simulink model "BTL"  (R2019b)
settings: Solver=FixedStepDiscrete  StartTime=0  StopTime=5  FixedStep=fixedStepSize  MaxStep=0.001  RelTol=1e-3  EnableMultiTasking=on
model workspace (MAT data in the model file):
  Occurrence.FaultRemote = 1
  Occurrence.FaultLow = 2
  Occurrence.FaultLow_2 = 3
  Occurrence.FaultModerate = 4
  Occurrence.FaultModerate_2 = 5
  Occurrence.FaultModerate_3 = 6
  Occurrence.FaultHigh = 7
  Occurrence.FaultHigh_2 = 8
  Occurrence.Tolerance = 9
  Occurrence.OK = 10
  Partitions.Last = ''
  Partitions.All = '*'
  Severity.OK = 0
  Severity.Warn = 1
  Severity.VeryMinor = 2
  Severity.Minor = 3
  Severity.VeryLow = 4
  Severity.Low = 5
  Severity.Moderate = 6
  Severity.High = 7
  Severity.VeryHigh = 8
  Severity.HazardousWithWarning = 9
  Severity.HazardousNoWarning = 10
  Severity.Error = 11
  Severity.ErrorFatal = 20
  block : handle (value not decoded)
  t = 0
  time = 0
undefined symbols (not defined in the file): BTL_evChangesTime, BTL_notAlwaysTime, BTL_notAlwaysTime2, BTL_preconditionGear, BTL_preconditionSpeedLim, BTL_preconditionSub1Value, BTL_preconditionSub1Value2, BTL_rpmLimit, BTL_sub1Value, BTL_sub1Value2, BTL_subsystem1_rpmLimit, BTL_subsystem1_speedLimit, fixedStepSize
libraries: simulink x1
settings Model: conn_id=-1  report_delay=1  Creator=aande176  LastModifiedBy=alex
settings SolverCC: AutoInsertRateTranBlk=on
settings DataIOCC: ExternalInput=[],CPSRSts__CPSRSts,[],[],[],[],[],[],[],LvTestSts__LvTestSts,IsgPwrLimMin__IsgPwrLimMin,[],IsgPwrLimMax__IsgPwrLimMax,TqAvlIntFromIfCpt__TqAvlIntFromIfCpt,[],[],[],[],[],TqAllwdInt__TqAllwdInt,[],[],[],[],[],[],[],HvBattUDynMaxLim__HvBattUDynMaxLim,[],HvBattUDynMinLim__HvBattUDynMinLim,[],InitCmpl__InitCmpl,[],[],[],[],[],[],[],[],[],[],[],HvTestSts__HvTestSts,[],[],[],IsgModReq__IsgModReq,[],[],[],[],[],[],[],[],[],[],[],[],[],[],[],[],[],EngSt1WdSts__EngSt1WdSts__IsUpdated,IsgSpdReq__IsgSpdReq__IsUpdated,IsgModReq__IsgModReq__IsUpdated,HvSysRlySts__HvSysRlySts__IsUpdated,HvSysRlySts_toController,[],[],[],[],ImobPrpsnAllwd__ImobPrpsnAllwd__dummy,[],[],[],[],ImobTurnOffAllwd__ImobTurnOffAllwd__dummy,[],[],[],No_GearEven,B_CloseClutchOdd,B_CloseClutchEven,[],[],[],B_EnableVSpAct,V_Vehicle_SetPoint_mps,[]  SaveFormat=StructureWithTime  SaveOutput=off  SaveTime=off  ReturnWorkspaceOutputs=off  SignalLoggingName=slunit_logdata
settings OptimizationCC: DefaultParameterBehavior=Inlined  ExpressionDepthLimit=2147483647  LifeSpan=Inf
settings DebuggingCC: RTPrefix=warning  AlgebraicLoopMsg=error  CheckSSInitialOutputMsg=off  SolverPrmCheckMsg=warning  IntegerOverflowMsg=none  ParameterPrecisionLossMsg=none  FcnCallInpInsideContextMsg=warning  BusObjectLabelMismatch=error  ModelReferenceDataLoggingMessage=none  StateNameClashWarn=warning  SFUnexpectedBacktrackingDiag=warning  SFNoUnconditionalDefaultTransitionDiag=warning  SFExecutionAtInitializationDiag=none  IntegerSaturationMsg=none  ArithmeticOperatorsInVariantConditions=warning
settings HardwareCC: ProdBitPerLong=64  ProdHWDeviceType=Intel->x86-64
settings ModelReferenceCC: UpdateModelReferenceTargets=AssumeUpToDate  PropagateSignalLabelsOutOfModel=off
settings SFSimCC: SimUseLocalCustomCode=off  SimGenImportedTypeDefs=on  CustomCodeUndefinedFunction=UseInterfaceOnly
settings RTWCC: RTWUseLocalCustomCode=off  RTWUseSimCustomCode=on
settings CodeAppCC: StateflowObjectComments=on
settings GRTTargetCC: TargetLangStandard=C89/C90 (ANSI)  GeneratePreprocessorConditionals=Disable all  CombineOutputUpdateFcns=off  MatFileLogging=off  GRTInterface=on
settings ConfigComp: CovScope=Subsystem  CovPath=RequirementsEvaluation/AvailableTorque  CovMetricSettings=dcw  CovHTMLOptions=-sRT=1 -aTS=1 -bRG=1 -bTC=1 -hTR=0 -nFC=0 -scm=1 -bcm=1 -xEv=0  CovHtmlReporting=on  CovSaveCumulativeToWorkspaceVar=on  CovSaveSingleToWorkspaceVar=on  CovExternalEMLEnable=off

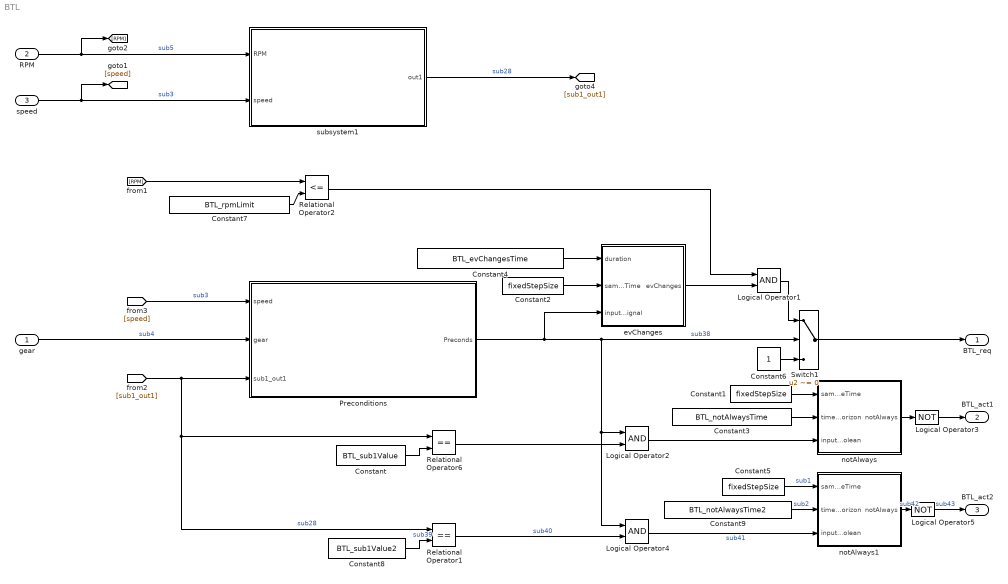
== system BTL ==
  gear : Inport  PortDimensions=1
  RPM : Inport  Port=2  PortDimensions=1
  speed : Inport  Port=3  PortDimensions=1
  Constant : Constant  Value=BTL_sub1Value
  Constant1 : Constant  Value=fixedStepSize
  Constant2 : Constant  Value=fixedStepSize
  Constant3 : Constant  Value=BTL_notAlwaysTime
  Constant4 : Constant  Value=BTL_evChangesTime
  Constant5 : Constant  Value=fixedStepSize
  Constant6 : Constant  OutDataTypeStr=boolean
  Constant7 : Constant  Value=BTL_rpmLimit
  Constant8 : Constant  Value=BTL_sub1Value2
  Constant9 : Constant  Value=BTL_notAlwaysTime2
  Logical Operator1 : Logic  AllPortsSameDT=off  OutDataTypeStr=boolean
  Logical Operator2 : Logic  AllPortsSameDT=off  OutDataTypeStr=boolean
  Logical Operator3 : Logic  Operator=NOT  AllPortsSameDT=off  OutDataTypeStr=boolean
  Logical Operator4 : Logic  AllPortsSameDT=off  OutDataTypeStr=boolean
  Logical Operator5 : Logic  Operator=NOT  AllPortsSameDT=off  OutDataTypeStr=boolean
  Preconditions : Subsystem
  Relational Operator1 : RelationalOperator  Operator===  OutDataTypeStr=boolean  RndMeth=Nearest
  Relational Operator2 : RelationalOperator  Operator=<=  OutDataTypeStr=boolean  RndMeth=Nearest
  Relational Operator6 : RelationalOperator  Operator===  OutDataTypeStr=boolean  RndMeth=Nearest
  Switch1 : Switch  Criteria=u2 ~= 0
  evChanges : Subsystem
      settings: CopyFcn=set_param(gcbh,'LinkStatus','none');
  notAlways : Subsystem
      settings: CopyFcn=set_param(gcbh,'LinkStatus','none');
  notAlways1 : Subsystem
      settings: CopyFcn=set_param(gcbh,'LinkStatus','none');
  subsystem1 : Subsystem
  BTL_req : Outport  OutDataTypeStr=boolean
  BTL_act1 : Outport  Port=2  OutDataTypeStr=boolean
  BTL_act2 : Outport  Port=3  OutDataTypeStr=boolean
  wires:
  RPM/1 -> subsystem1/1(RPM), [RPM]  "sub5"
  speed/1 -> [speed], subsystem1/2(speed)  "sub3"
  subsystem1/1(out1) -> [sub1_out1]  "sub28"
  Logical Operator5/1 -> BTL_act2/1  "sub43"
  Constant7/1 -> Relational Operator2/2
  Relational Operator2/1 -> Logical Operator1/1
  Constant1/1 -> notAlways/1(sampleTime)
  Constant8/1 -> Relational Operator1/2  "sub39"
  Relational Operator1/1 -> Logical Operator4/2  "sub40"
  [sub1_out1] -> Relational Operator1/1, Relational Operator6/1, Preconditions/3(sub1_out1)  "sub28"
  notAlways1/1(notAlways) -> Logical Operator5/1  "sub42"
  Constant5/1 -> notAlways1/1(sampleTime)  "sub1"
  Constant2/1 -> evChanges/2(sampleTime)
  Logical Operator1/1 -> Switch1/1
  Constant9/1 -> notAlways1/2(timeHorizon)  "sub2"
  Logical Operator3/1 -> BTL_act1/1
  [speed] -> Preconditions/1(speed)  "sub3"
  Constant6/1 -> Switch1/3
  Logical Operator2/1 -> notAlways/3(inputBoolean)
  Relational Operator6/1 -> Logical Operator2/2
  Constant3/1 -> notAlways/2(timeHorizon)
  Constant/1 -> Relational Operator6/2
  Logical Operator4/1 -> notAlways1/3(inputBoolean)  "sub41"
  Preconditions/1(Preconds) -> evChanges/3(inputSignal), Switch1/2, Logical Operator2/1, Logical Operator4/1  "sub38"
  gear/1 -> Preconditions/2(gear)  "sub4"
  Constant4/1 -> evChanges/1(duration)
  evChanges/1(evChanges) -> Logical Operator1/2
  Switch1/1 -> BTL_req/1
  notAlways/1(notAlways) -> Logical Operator3/1
  [RPM] -> Relational Operator2/1

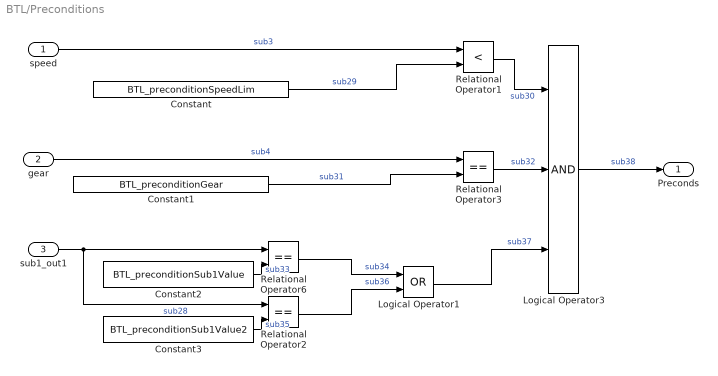
== system BTL/Preconditions ==
  speed : Inport
  gear : Inport  Port=2
  sub1_out1 : Inport  Port=3
  Constant : Constant  Value=BTL_preconditionSpeedLim
  Constant1 : Constant  Value=BTL_preconditionGear
  Constant2 : Constant  Value=BTL_preconditionSub1Value
  Constant3 : Constant  Value=BTL_preconditionSub1Value2
  Logical Operator1 : Logic  Operator=OR  AllPortsSameDT=off  OutDataTypeStr=boolean
  Logical Operator3 : Logic  Inputs=3  AllPortsSameDT=off  OutDataTypeStr=boolean
  Relational Operator1 : RelationalOperator  Operator=<  OutDataTypeStr=boolean  RndMeth=Nearest
  Relational Operator2 : RelationalOperator  Operator===  OutDataTypeStr=boolean  RndMeth=Nearest
  Relational Operator3 : RelationalOperator  Operator===  OutDataTypeStr=boolean  RndMeth=Nearest
  Relational Operator6 : RelationalOperator  Operator===  OutDataTypeStr=boolean  RndMeth=Nearest
  Preconds : Outport
  wires:
  speed/1 -> Relational Operator1/1  "sub3"
  Constant/1 -> Relational Operator1/2  "sub29"
  gear/1 -> Relational Operator3/1  "sub4"
  Relational Operator3/1 -> Logical Operator3/2  "sub32"
  Relational Operator1/1 -> Logical Operator3/1  "sub30"
  Logical Operator1/1 -> Logical Operator3/3  "sub37"
  Logical Operator3/1 -> Preconds/1  "sub38"
  sub1_out1/1 -> Relational Operator2/1, Relational Operator6/1  "sub28"
  Constant2/1 -> Relational Operator6/2  "sub33"
  Constant3/1 -> Relational Operator2/2  "sub35"
  Relational Operator6/1 -> Logical Operator1/1  "sub34"
  Relational Operator2/1 -> Logical Operator1/2  "sub36"
  Constant1/1 -> Relational Operator3/2  "sub31"

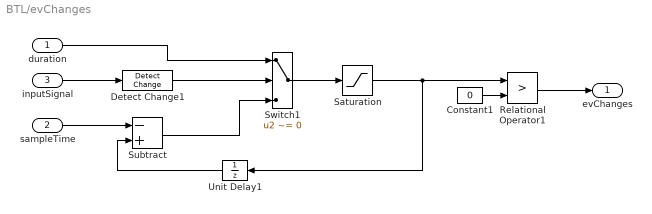
== system BTL/evChanges ==
  duration : Inport
  sampleTime : Inport  Port=2
  inputSignal : Inport  Port=3
  Constant1 : Constant  Value=0
  Detect Change1 : simulink/Logic and Bit Operations/Detect Change  vinit=0  OutDataTypeStr=boolean
  Relational Operator1 : RelationalOperator  Operator=>  OutDataTypeStr=boolean  RndMeth=Nearest
  Saturation : Saturate  UpperLimit=Inf  LowerLimit=0
  Subtract : Sum  Inputs=-+
  Switch1 : Switch  Criteria=u2 ~= 0
  Unit Delay1 : UnitDelay  SampleTime=-1  HasFrameUpgradeWarning=on
  evChanges : Outport  VectorParamsAs1DForOutWhenUnconnected=off
  wires:
  Detect Change1/1 -> Switch1/2
  duration/1 -> Switch1/1
  Switch1/1 -> Saturation/1
  inputSignal/1 -> Detect Change1/1
  Constant1/1 -> Relational Operator1/2
  Subtract/1 -> Switch1/3
  Saturation/1 -> Relational Operator1/1, Unit Delay1/1
  Unit Delay1/1 -> Subtract/2
  Relational Operator1/1 -> evChanges/1
  sampleTime/1 -> Subtract/1

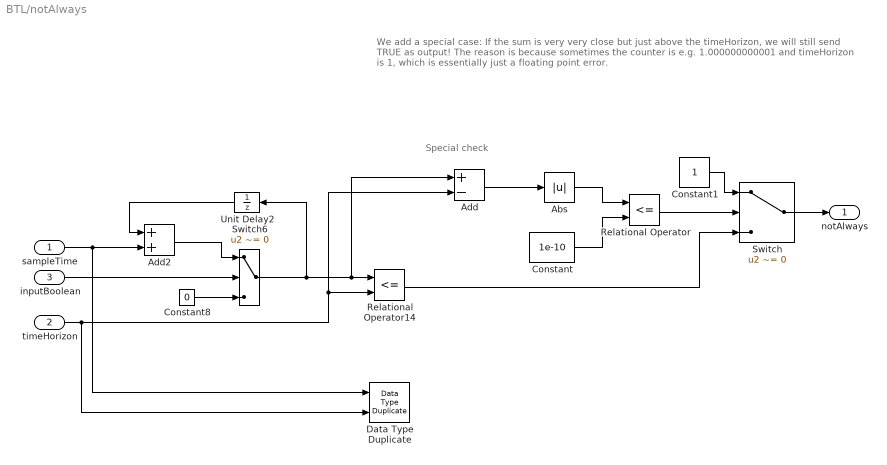
== system BTL/notAlways ==
  note: Special check
  note: We add a special case:
      | If the sum is very very close but just above the timeHorizon, we will still send TRUE as output!
      |
      | The reason is because sometimes the counter is e.g. 1.000000000001 and timeHorizon is 1, which is essentially just a floating point error.
  sampleTime : Inport
  timeHorizon : Inport  Port=2
  inputBoolean : Inport  Port=3
  Abs : Abs
  Add : Sum  Inputs=+-
  Add2 : Sum
  Constant : Constant  Value=1e-10
  Constant1 : Constant  OutDataTypeStr=boolean
  Constant8 : Constant  Value=0  OutDataTypeStr=Inherit: Inherit via back propagation
  Data Type Duplicate : DataTypeDuplicate
  Relational Operator : RelationalOperator  Operator=<=  OutDataTypeStr=boolean  RndMeth=Simplest
  Relational Operator14 : RelationalOperator  Operator=<=  OutDataTypeStr=boolean  RndMeth=Nearest
  Switch : Switch  Criteria=u2 ~= 0
  Switch6 : Switch  Criteria=u2 ~= 0
  Unit Delay2 : UnitDelay  SampleTime=-1  HasFrameUpgradeWarning=on
  notAlways : Outport  VectorParamsAs1DForOutWhenUnconnected=off
  wires:
  Switch6/1 -> Add/1, Relational Operator14/1, Unit Delay2/1
  timeHorizon/1 -> Add/2, Relational Operator14/2, Data Type Duplicate/2
  Relational Operator14/1 -> Switch/3
  Unit Delay2/1 -> Add2/1
  Add2/1 -> Switch6/1
  sampleTime/1 -> Add2/2, Data Type Duplicate/1
  Constant8/1 -> Switch6/3
  inputBoolean/1 -> Switch6/2
  Add/1 -> Abs/1
  Abs/1 -> Relational Operator/1
  Constant/1 -> Relational Operator/2
  Relational Operator/1 -> Switch/2
  Constant1/1 -> Switch/1
  Switch/1 -> notAlways/1

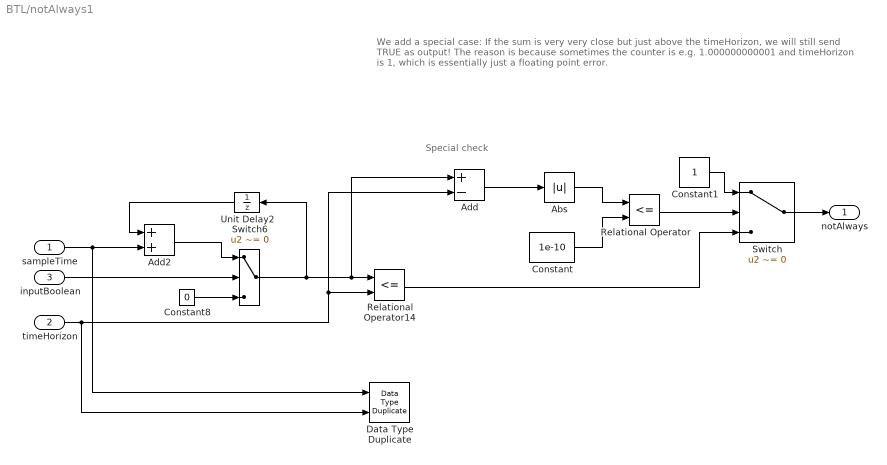
== system BTL/notAlways1 ==
  note: Special check
  note: We add a special case:
      | If the sum is very very close but just above the timeHorizon, we will still send TRUE as output!
      |
      | The reason is because sometimes the counter is e.g. 1.000000000001 and timeHorizon is 1, which is essentially just a floating point error.
  sampleTime : Inport
  timeHorizon : Inport  Port=2
  inputBoolean : Inport  Port=3
  Abs : Abs
  Add : Sum  Inputs=+-
  Add2 : Sum
  Constant : Constant  Value=1e-10
  Constant1 : Constant  OutDataTypeStr=boolean
  Constant8 : Constant  Value=0  OutDataTypeStr=Inherit: Inherit via back propagation
  Data Type Duplicate : DataTypeDuplicate
  Relational Operator : RelationalOperator  Operator=<=  OutDataTypeStr=boolean  RndMeth=Simplest
  Relational Operator14 : RelationalOperator  Operator=<=  OutDataTypeStr=boolean  RndMeth=Nearest
  Switch : Switch  Criteria=u2 ~= 0
  Switch6 : Switch  Criteria=u2 ~= 0
  Unit Delay2 : UnitDelay  SampleTime=-1  HasFrameUpgradeWarning=on
  notAlways : Outport  VectorParamsAs1DForOutWhenUnconnected=off
  wires:
  Switch6/1 -> Add/1, Relational Operator14/1, Unit Delay2/1
  timeHorizon/1 -> Add/2, Relational Operator14/2, Data Type Duplicate/2
  Relational Operator14/1 -> Switch/3
  Unit Delay2/1 -> Add2/1
  Add2/1 -> Switch6/1
  sampleTime/1 -> Add2/2, Data Type Duplicate/1
  Constant8/1 -> Switch6/3
  inputBoolean/1 -> Switch6/2
  Add/1 -> Abs/1
  Abs/1 -> Relational Operator/1
  Constant/1 -> Relational Operator/2
  Relational Operator/1 -> Switch/2
  Constant1/1 -> Switch/1
  Switch/1 -> notAlways/1

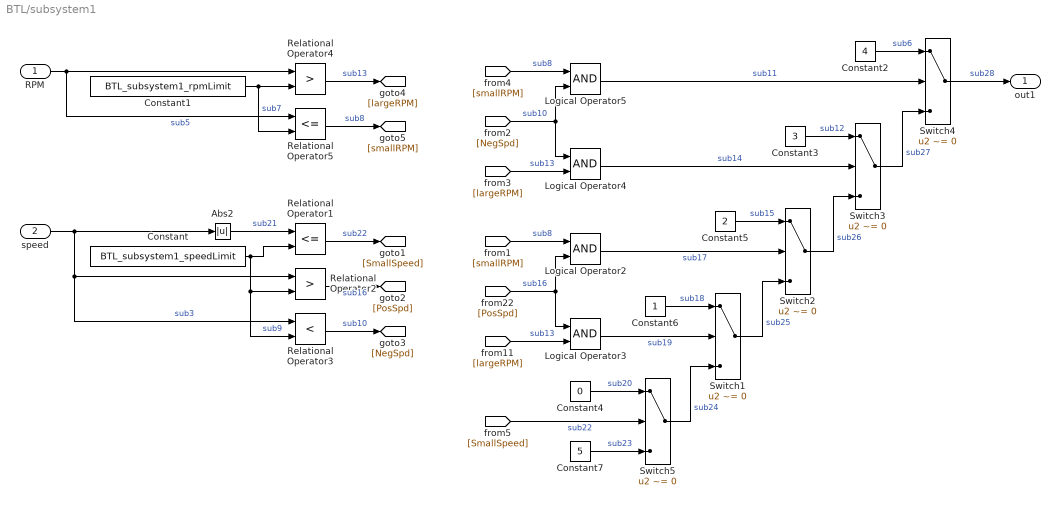
== system BTL/subsystem1 ==
  RPM : Inport
  speed : Inport  Port=2
  Abs2 : Abs
  Constant : Constant  Value=BTL_subsystem1_speedLimit
  Constant1 : Constant  Value=BTL_subsystem1_rpmLimit
  Constant2 : Constant  Value=4
  Constant3 : Constant  Value=3
  Constant4 : Constant  Value=0
  Constant5 : Constant  Value=2
  Constant6 : Constant
  Constant7 : Constant  Value=5
  Logical Operator{2..5} (4 alike) : Logic  AllPortsSameDT=off  OutDataTypeStr=boolean
  Relational Operator1 : RelationalOperator  Operator=<=  OutDataTypeStr=boolean  RndMeth=Nearest
  Relational Operator2 : RelationalOperator  Operator=>  OutDataTypeStr=boolean  RndMeth=Nearest
  Relational Operator3 : RelationalOperator  Operator=<  OutDataTypeStr=boolean  RndMeth=Nearest
  Relational Operator4 : RelationalOperator  Operator=>  OutDataTypeStr=boolean  RndMeth=Nearest
  Relational Operator5 : RelationalOperator  Operator=<=  OutDataTypeStr=boolean  RndMeth=Nearest
  Switch{1..5} (5 alike) : Switch  Criteria=u2 ~= 0
  out1 : Outport
  wires:
  Relational Operator1/1 -> [SmallSpeed]  "sub22"
  RPM/1 -> Relational Operator5/1, Relational Operator4/1  "sub5"
  speed/1 -> Abs2/1, Relational Operator2/1, Relational Operator3/1  "sub3"
  Relational Operator2/1 -> [PosSpd]  "sub16"
  Relational Operator3/1 -> [NegSpd]  "sub10"
  [PosSpd] -> Logical Operator3/1, Logical Operator2/2  "sub16"
  [smallRPM] -> Logical Operator2/1  "sub8"
  Relational Operator4/1 -> [largeRPM]  "sub13"
  Relational Operator5/1 -> [smallRPM]  "sub8"
  Constant/1 -> Relational Operator3/2, Relational Operator2/2, Relational Operator1/2  "sub9"
  [largeRPM] -> Logical Operator3/2  "sub13"
  [largeRPM] -> Logical Operator4/2  "sub13"
  [smallRPM] -> Logical Operator5/1  "sub8"
  [NegSpd] -> Logical Operator5/2, Logical Operator4/1  "sub10"
  Logical Operator3/1 -> Switch1/2  "sub19"
  Logical Operator2/1 -> Switch2/2  "sub17"
  Switch1/1 -> Switch2/3  "sub25"
  Switch2/1 -> Switch3/3  "sub26"
  Logical Operator4/1 -> Switch3/2  "sub14"
  Logical Operator5/1 -> Switch4/2  "sub11"
  Constant6/1 -> Switch1/1  "sub18"
  Constant5/1 -> Switch2/1  "sub15"
  Constant3/1 -> Switch3/1  "sub12"
  Constant2/1 -> Switch4/1  "sub6"
  Switch3/1 -> Switch4/3  "sub27"
  [SmallSpeed] -> Switch5/2  "sub22"
  Switch5/1 -> Switch1/3  "sub24"
  Constant4/1 -> Switch5/1  "sub20"
  Constant7/1 -> Switch5/3  "sub23"
  Switch4/1 -> out1/1  "sub28"
  Abs2/1 -> Relational Operator1/1  "sub21"
  Constant1/1 -> Relational Operator5/2, Relational Operator4/2  "sub7"
